simulink model "fft_core2"  (R2013a)
settings: Solver=VariableStepDiscrete  SolverMode=SingleTasking  StartTime=0.0  StopTime=4096*(4096/16) + 10000  RelTol=1e-3
undefined symbols (not defined in the file or in its folder): A, B, C, PCIN, xlipgetpartsetting
libraries: xbsIndex_r4 x20912, casper_library_misc x110, casper_library_reorder x8, casper_library_delays x4, xbsReplacements_r4 x2
(part 1 of 187)
settings Model: Creator=rprimian  LastModifiedBy=jack
settings Model: ModifiedComment=|
  | jack -- Wed Jan 14 18:05:02 2015 -- Version 1.207
  | resynthed
settings Model: ModifiedHistory=|
  | jack -- Wed Jan 14 18:05:02 2015 -- Version 1.207
  | resynthed
  | 
  | jack -- Wed Jan 14 17:38:02 2015 -- Version 1.206
  | 
  | 
  | jack -- Wed Jan 14 17:23:08 2015 -- Version 1.205
  | fanout write address / buf sel signals in unscrambler
  | 
  | jack -- Sun Jan 11 19:22:28 2015 -- Version 1.204
  | generated (lc off, equiv reg removal no)
  | 
  | jack -- Sun Jan 11 18:52:11 2015 -- Version 1.203
  | manual fanout control fft_stage_1 sync input
  | 
  | jack -- Sun Jan 11 12:56:59 2015 -- Version 1.202
  | regened
  | 
  | jack -- Sun Jan 11 12:38:07 2015 -- Version 1.201
  | manual fanout control between direct butterfly 2_0 and 3_0 sync
  | 
  | jack -- Sun Jan 11 12:11:23 2015 -- Version 1.200
  | implement counter in fft stage 1 as behavioural hdl
  | 
  | jack -- Fri Jan 09 10:07:59 2015 -- Version 1.199
  | generated
  | 
  | jack -- Wed Jan 07 15:06:47 2015 -- Version 1.198
  | xlupdatemodel for 14.7
  | 
  | jack -- Wed Jan 07 14:01:30 2015 -- Version 1.197
  | change butterfly max fanout to 2
  | 
  | jack -- Sun Dec 07 16:26:38 2014 -- Version 1.196
  | removed core delay attribute in coeff of butterfly 2_0
  | 
  | jack -- Thu Dec 04 23:51:50 2014 -- Version 1.195
  | change delay in butterfly 2-0 coeffgen to be core
  | 
  | jack -- Thu Dec 04 21:24:02 2014 -- Version 1.194
  | gen'd
  | 
  | jack -- Thu Dec 04 21:00:43 2014 -- Version 1.193
  | multiplexer latency=1
  | 
  | jack -- Wed Dec 03 18:09:45 2014 -- Version 1.192
  | regenerated
  | 
  | jack -- Wed Dec 03 15:44:47 2014 -- Version 1.191
  | regenerated
  | 
  | jack -- Wed Dec 03 14:18:08 2014 -- Version 1.190
  | added in descramble
  | 
  | jack -- Wed Dec 03 00:08:02 2014 -- Version 1.189
  | added back in butterfly2-0 sync out fanout regs
  | 
  | jack -- Tue Dec 02 21:40:43 2014 -- Version 1.188
  | all cast latency to 2 in fft direct
  | 
  | jack -- Tue Dec 02 17:31:35 2014 -- Version 1.187
  | remove input latency
  | 
  | jack -- Tue Dec 02 17:27:04 2014 -- Version 1.186
  | forgot to change hilbert addsubs to 'complex'
  | 
  | jack -- Tue Dec 02 17:16:05 2014 -- Version 1.185
  | ready to regenerate after fixing dsp complex adders and cmult latencies
  | 
  | jack -- Fri Nov 28 18:02:27 2014 -- Version 1.184
  | reduced fanout registering in cmult of butterfly 0_0 twiddle
  | 
  | jack -- Fri Nov 28 17:54:11 2014 -- Version 1.183
  | delay cores in biplex descramble reorder data delays
  | 
  | jack -- Fri Nov 28 17:51:35 2014 -- Version 1.182
  | implement sync delays in butterfly 3_0, 3_1 twiddles as cores
  | 
  | jack -- Fri Nov 28 15:14:09 2014 -- Version 1.181
  | regenerated
  | 
  | jack -- Fri Nov 28 14:47:31 2014 -- Version 1.180
  | update diagram
  | 
  | jack -- Fri Nov 28 14:11:29 2014 -- Version 1.179
  | 
  | syntax fix
  | 
  | jack -- Fri Nov 28 13:12:47 2014 -- Version 1.178
  | 
  | changed cast latency to 2 in both parts of FFT
  | 
  | jack -- Thu Nov 27 18:11:31 2014 -- Version 1.177
  | regenerated
  | 
  | jack -- Thu Nov 27 17:24:07 2014 -- Version 1.176
  | implement dsync 1 and dsync2 delays in fft stage 1 as cores (fanout control)
  | 
  | jack -- Wed Oct 29 13:45:38 2014 -- Version 1.175
  | regenerated in correct location
  | 
  | jack -- Wed Oct 29 08:59:41 2014 -- Version 1.174
  | wastn't generating to fft_core2.ngc! Last version of that file was from 26th oct 1159.
  | 
  | jack -- Wed Oct 29 02:01:36 2014 -- Version 1.173
  | 
  | 
  | jack -- Wed Oct 29 01:59:56 2014 -- Version 1.172
  | regenerated
  | 
  | jack -- Wed Oct 29 01:21:04 2014 -- Version 1.171
  | manual fanout control between direct butterfly 2_0 and 3_0 sync
  | 
  | jack -- Tue Oct 28 19:29:52 2014 -- Version 1.170
  | change latency between biplex and direct to 0
  | 
  | jack -- Mon Oct 27 18:43:05 2014 -- Version 1.169
  | added comment about manually changing hiltert addsubs to use dsp
  | 
  | jack -- Mon Oct 27 18:42:18 2014 -- Version 1.168
  | changed casts outside twiddles to latency 2, then redid manual changes
  | 
  | jack -- Sun Oct 26 11:03:45 2014 -- Version 1.167
  | dupe core for some experimenting :)
  | 
  | jack -- Sun Oct 26 10:45:07 2014 -- Version 1.166
  | delay on data-b in butterfly0_0 cmult changed to core
  | 
  | jack -- Sun Oct 26 10:25:39 2014 -- Version 1.165
  | latency between biplkex and direct back to 1
  | 
  | jack -- Sat Oct 25 15:09:40 2014 -- Version 1.164
  | regenerated
  | 
  | jack -- Sat Oct 25 14:36:46 2014 -- Version 1.163
  | do back to fabric adders in hilberts
  | 
  | jack -- Fri Oct 24 23:13:10 2014 -- Version 1.162
  | changed hilbert blocks in bi_real_unscr_4x to dsp implementation
  | 
  | jack -- Fri Oct 24 14:47:43 2014 -- Version 1.161
  | increased latency between biplex and direct fft to 2
  | 
  | jack -- Tue Oct 21 15:26:40 2014 -- Version 1.160
  | regenerated
  | 
  | jack -- Tue Oct 21 14:20:46 2014 -- Version 1.159
  | 
  | notes reminding me what to manually add if the FFT needs autmatically redrawing!
  | 
  | jack -- Tue Oct 21 14:18:23 2014 -- Version 1.158
  | 
  | made reorders in descramble not asynchronous
  | 
  | jack -- Tue Oct 21 11:02:41 2014 -- Version 1.157
  | 
  | 
  | jack -- Tue Oct 21 10:46:08 2014 -- Version 1.156
  | regenerated, after changing twiddle init script to reduce the number of fanout registers in cmults -- now it only puts a register where there is real fanout.
  | 
  | jack -- Tue Oct 21 09:44:16 2014 -- Version 1.155
  | 
  | 
  | jack -- Tue Oct 21 09:43:06 2014 -- Version 1.154
  | set dmux0 in fft_stage1 to use core delay (rather than behavioural HDL)
  | 
  | jack -- Mon Oct 20 17:21:54 2014 -- Version 1.153
  | generated
  | 
  | jack -- Mon Oct 20 15:57:34 2014 -- Version 1.152
  | remove channel order descramble
  | 
  | jack -- Mon Oct 20 15:47:10 2014 -- Version 1.150
  | 
  | change fft unscrambled to double buffer, and add some fanout delay. NOTE: this change requires manual setting of the FFT unscrambler block
  | 
  | jack -- Mon Oct 20 15:48:32 2014 -- Version 1.150
  | don't bother unscrambling
  | 
  | jack -- Mon Oct 20 10:32:55 2014 -- Version 1.149
  |  change data delays in bram_delay blocks to be inmplemented as cores. Reduce fanout delay from (max(1, log2(number_of_brams)) to max(1, log2(number_of_brams / max fanout))
  | 
  | jack -- Sun Oct 19 18:00:08 2014 -- Version 1.148
  | change add latency in biplex unscramble to 3, perform casts in xilinx cast blocks
  | 
  | jack -- Fri Oct 17 15:52:50 2014 -- Version 1.147
  | move adders everywhere to dsp. casts everywhere to logic
  | 
  | jack -- Wed Oct 15 14:23:41 2014 -- Version 1.146
  | regenerated with fft direct adders in dsps (one dsp per 2 adds / 2subs)
  | 
  | jack -- Wed Oct 15 11:45:00 2014 -- Version 1.145
  | 
  | changed fft direct to do adds in dsp. NOTE: This requires setting manually below the top level block!
  | 
  | jack -- Tue Oct 14 16:11:01 2014 -- Version 1.144
  | 
  | 
  | jack -- Mon Oct 13 18:35:49 2014 -- Version 1.143
  | redraw with 1 cycle latency on overflow comparators in butterflies
  | 
  | jack -- Thu Oct 09 14:59:23 2014 -- Version 1.142
  | regenerated
  | 
  | jack -- Thu Oct 09 14:39:22 2014 -- Version 1.141
  | replaced cmults with explicit dsp48 cmults using macros
  | 
  | jack -- Wed Oct 08 16:18:36 2014 -- Version 1.140
  | 
  | bram latency increase to 4 (only really necessary for the last stage of the dirrect butterflies, where there is no fanout and inadequate latency to go from bram to dsp in one clock)
  | 
  | jack -- Wed Oct 08 09:37:16 2014 -- Version 1.139
  | regenerated
  | 
  | jack -- Tue Oct 07 20:30:28 2014 -- Version 1.138
  | 
  | regnerated with cosin vanilla blocks in coefficient generators
  | 
  | jack -- Thu Sep 25 12:10:32 2014 -- Version 1.137
  | 
  | 
  | jack -- Thu Sep 25 12:10:01 2014 -- Version 1.136
  | 
  | 
  | jack -- Thu Sep 25 11:52:10 2014 -- Version 1.135
  | 
  | 
  | jack -- Thu Sep 25 10:42:48 2014 -- Version 1.134
  | 
  | manually changed the fft_unscrambler/reoder block.
  | -- double buffer
  | -- bram latency 3 (was 2)
  | -- manual drawing to fanout delay_sel and wr_addr signals
  | 
  | jack -- Tue Sep 23 10:03:49 2014 -- Version 1.133
  | 
  | synthesized
  | 
  | jack -- Mon Sep 22 14:47:38 2014 -- Version 1.132
  | changed adder implementation (in draw script) of butterfly adds to soft core (unless dsp chosen). Previously was behavioural
  | 
  | jack -- Sat Sep 20 12:31:03 2014 -- Version 1.131
  | 
  | compile (L shape constraints) failled spectacularly with dsp cast latency 2. Changed latency to 3.
  | Also lowered bram latency to 3
  | 
  | jack -- Fri Sep 19 18:08:32 2014 -- Version 1.130
  | regenerated
  | 
  | jack -- Fri Sep 19 15:47:10 2014 -- Version 1.129
  | 
  | changed cast latency in twiddles (which use dsps) to 2
  | 
  | jack -- Mon Sep 08 17:31:18 2014 -- Version 1.128
  | 
  | manual pipelining for fft_stage1
  | 
  | jack -- Tue Jun 03 23:16:33 2014 -- Version 1.127
  | 
  | 
  | jack -- Tue Jun 03 20:04:26 2014 -- Version 1.126
  | 
  | 
  | jack -- Mon Jun 02 09:04:22 2014 -- Version 1.125
  | pipelined overflow flag chain in fft direct
  | 
  | jack -- Mon Jun 02 07:25:10 2014 -- Version 1.124
  | manually added register stages to fft biplex stages 1 and 2.
  | changed convert latency in butterflies (dsp-based) to 4
  | 
  | jack -- Sat Mar 22 14:42:09 2014 -- Version 1.123
  | changed fft descramble to not use double buffering.
  | 
  | jack -- Fri Mar 21 17:47:36 2014 -- Version 1.122
  | changed reorder brams to optimize for speed
  | 
  | jack -- Sun Mar 16 21:17:26 2014 -- Version 1.121
  | fanout control on unscramblers
  | 
  | jack -- Thu Feb 20 17:09:35 2014 -- Version 1.120
  | changed bram latency in descramble to 3 to avoid using srls. will add more pipelineing in main model
  | 
  | jack -- Wed Feb 19 19:33:34 2014 -- Version 1.119
  | generated
  | 
  | jack -- Wed Feb 19 18:32:15 2014 -- Version 1.118
  | put bthe descramble back. changed max_fanout to 2
  | 
  | jack -- Fri Feb 14 17:39:39 2014 -- Version 1.117
  | 
  | 
  | jack -- Fri Feb 14 17:34:13 2014 -- Version 1.116
  | 
  | changed add latency to 3 (was 2) outside twiddles
  | 
  | jack -- Thu Feb 13 18:32:54 2014 -- Version 1.115
  | 
  | Easy timing fix to descramble -- don't bother doing it!
  | 
  | jack -- Thu Feb 13 18:11:13 2014 -- Version 1.114
  | 
  | turned down descramble bram latency to 3
  | 
  | jack -- Tue Feb 11 21:59:13 2014 -- Version 1.113
  | synth'd
  | 
  | jack -- Tue Feb 11 19:54:11 2014 -- Version 1.112
  | 
  | Changed brams in descramble reorder to optimize for speed
  | 
  | jack -- Tue Feb 11 17:12:22 2014 -- Version 1.111
  | 
  | Regenerated
  | 
  | jack -- Tue Feb 11 17:11:17 2014 -- Version 1.110
  | 
  | Changed reorder in fft_unscrambler to use double buffering, and fanout delay of 1
  | 
  | jack -- Tue Feb 04 10:57:01 2014 -- Version 1.109
  | regenerated
  | 
  | jack -- Mon Feb 03 17:18:37 2014 -- Version 1.108
  | change shift schedule
  | 
  | jack -- Mon Feb 03 13:02:14 2014 -- Version 1.107
  | complexified simulation outputs
  | 
  | jack -- Mon Feb 03 10:41:09 2014 -- Version 1.106
  | 
  | 
  | jack -- Mon Feb 03 10:39:20 2014 -- Version 1.105
  | 
  | 
  | jack -- Mon Feb 03 10:36:49 2014 -- Version 1.104
  | 
  | Added simulation model --  a series of 1 cycle impulsesat each of 4096 positions
  | 
  | jack -- Mon Feb 03 10:22:35 2014 -- Version 1.103
  | 
  | 
  | jack -- Sat Feb 01 23:42:24 2014 -- Version 1.102
  | Increased bram latency to 4
  | 
  | jack -- Fri Jan 31 22:38:23 2014 -- Version 1.101
  | 
  | Bug in fft_stage_n_init when using slice-based delays. A fanout delay was being compensated for on the sync lines, but did not actually appear on the data lines. Fixed this in the init script -- going for a recompile.
  | 
  | jack -- Fri Jan 31 17:45:46 2014 -- Version 1.100
  | 
  | Added a scope to input
  | 
  | jack -- Wed Jan 29 17:53:39 2014 -- Version 1.99
  | 
  | Generated core
  | 
  | jack -- Wed Jan 29 17:04:46 2014 -- Version 1.98
  | 
  | Changed max fanout to 1
  | 
  | jack -- Wed Jan 29 13:58:52 2014 -- Version 1.97
  | 
  | Changed delay blocks to attach constant 1 to we inputs. Before it was a constant going through a fanout/reinterpret/slice, which doesn't optimize away properly.
  | 
  | reverted to sampled constant one's. Failed compile with unsampled constants.
  | 
  | 
  | 
  | Recompile after setting we constants to be unsampled.
  | Previous compiles caused timing errors due to we fanout even though the signal is static
settings DataIOCC: SignalLoggingSaveFormat=ModelDataLogs
settings OptimizationCC: InlineParams=on  ExpressionDepthLimit=2147483647
settings DebuggingCC: FcnCallInpInsideContextMsg=UseLocalSettings
settings GRTTargetCC: CombineOutputUpdateFcns=off  GRTInterface=on

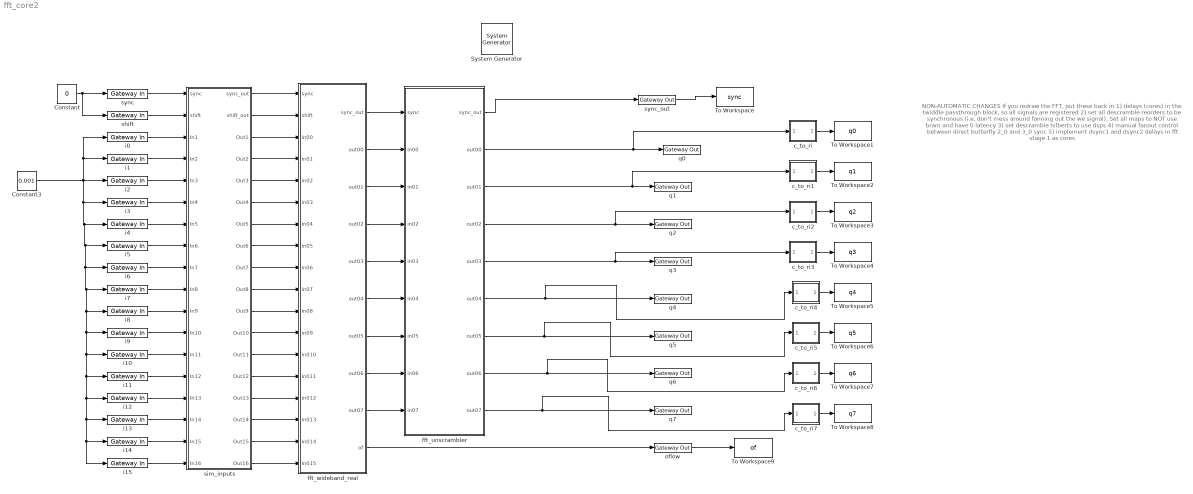
== system fft_core2 ==
  note: NON-AUTOMATIC CHANGES
      |
      | If you redraw the FFT, put these back in
      |
      | 1) delays (cores) in the twiddle passthrough block, so all signals are registered
      |
      | 2) set all descramble reorders to be synchronous (i.e, don't mess around fanning
      | out the we signal). Set all maps to NOT use bram and have 0 latency
      |
      | 3) set descramble hilberts to use dsps
      |
      | 4) manual fanout control between direct butterfly 2_0 and 3_0 sync
      |
      | 5) implement dsync1 and dsync2 delays in fft stage 1 as cores
  " System Generator" : xbsIndex_r4/ System Generator  Tag=genX  xilinxfamily=virtex6  part=xc6vsx475t  speed=-1  package=ff1759  synthesis_tool=XST  clock_wrapper=Clock Enables  directory=./fft_core2  proj_type=Project Navigator  Synth_file=XST Defaults  Impl_file=ISE Defaults  testbench=off  simulink_period=1  sysclk_period=3  dcm_input_clock_period=100  incr_netlist=off  trim_vbits=Everywhere in SubSystem  dbl_ovrd=According to Block Masks  core_generation=According to Block Masks  run_coregen=off  deprecated_control=off  eval_field=0  block_type=sysgen
      settings: block_version=11.4
  Constant : Constant  Value=0
  Constant3 : Constant  Value=0.001
  To Workspace : ToWorkspace  VariableName=sync  SampleTime=-1  SaveFormat=Timeseries
  To Workspace1 : ToWorkspace  VariableName=q0  SampleTime=-1  SaveFormat=Timeseries
  To Workspace2 : ToWorkspace  VariableName=q1  SampleTime=-1  SaveFormat=Timeseries
  To Workspace3 : ToWorkspace  VariableName=q2  SampleTime=-1  SaveFormat=Timeseries
  To Workspace4 : ToWorkspace  VariableName=q3  SampleTime=-1  SaveFormat=Timeseries
  To Workspace5 : ToWorkspace  VariableName=q4  SampleTime=-1  SaveFormat=Timeseries
  To Workspace6 : ToWorkspace  VariableName=q5  SampleTime=-1  SaveFormat=Timeseries
  To Workspace7 : ToWorkspace  VariableName=q6  SampleTime=-1  SaveFormat=Timeseries
  To Workspace8 : ToWorkspace  VariableName=q7  SampleTime=-1  SaveFormat=Timeseries
  To Workspace9 : ToWorkspace  VariableName=of  SampleTime=-1  SaveFormat=Timeseries
  c_to_ri : Subsystem
  c_to_ri1 : Subsystem
  c_to_ri2 : Subsystem
  c_to_ri3 : Subsystem
  c_to_ri4 : Subsystem
  c_to_ri5 : Subsystem
  c_to_ri6 : Subsystem
  c_to_ri7 : Subsystem
  fft_unscrambler : Subsystem  AncestorBlock=casper_library_ffts/fft_unscrambler  mask(fft_unscrambler){n_streams=1, FFTSize=11, n_inputs=3, n_bits_in=18, bram_latency=3, coeffs_bit_limit=8, async=off}
      mask prompts: n_streams "Number of simultaneous streams"; FFTSize "Size of FFT: (2^?)"; n_inputs "Number of simultaneous inputs: (2^?)"; n_bits_in "Input bit width"; bram_latency "BRAM Latency"; coeffs_bit_limit "Number bits above which to store map coefficients in BRAM (2^? bits)"; async "Asynchronous operation"
      mask init:
      | fft_unscrambler_init(gcb, ...
      |     'n_streams', n_streams, ...
      |     'FFTSize',FFTSize, ... 
      |     'n_inputs', n_inputs, ...
      |     'n_bits_in', n_bits_in, ...
      |     'bram_latency', bram_latency, ...
      |     'coeffs_bit_limit', coeffs_bit_limit, ...
      |     'async', async);
      settings: AttributesFormatString=FFTSize=11, n_inputs=3
  fft_wideband_real : Subsystem  Tag=casper:fft_wideband_real  AncestorBlock=casper_library_ffts/fft_wideband_real  mask(fft_wideband_real){n_streams=1, FFTSize=12, n_inputs=4, input_bit_width=18, bin_pt_in=17, coeff_bit_width=18, unscramble=off, async=off, add_latency=2, add_latency_twiddles=1, mult_latency=3, bram_latency=3, conv_latency=1, conv_latency_twiddles=1, input_latency=0, biplex_direct_latency=0, quantization=Round  (unbiased: +/- Inf), overflow=Wrap, delays_bit_limit=8, coeffs_bit_limit=8, coeff_sharing=off, coeff_decimation=off, coeff_generation=off, cal_bits=1, n_bits_rotation=25, mult_spec=1, max_fanout=4, bitgrowth=off, max_bits=19, hardcode_shifts=off, shift_schedule=[], dsp48_adders=on, conv_imp_twiddles=Xilinx Cast Block, conv_imp=Xilinx Cast Block}
      mask prompts: n_streams "Number simultaneous streams"; FFTSize "Size of FFT: (2^? pts)"; n_inputs "Number of Simultaneous Inputs: (2^?)"; input_bit_width "Input Bit Width"; bin_pt_in "Input binary point"; coeff_bit_width "Coefficient Bit Width"; unscramble "Unscramble output (ie, put channels in canonical order)"; async "Asynchronous operation"; add_latency "Add Latency"; add_latency_twiddles "Add Latency (in twiddles)"; mult_latency "Mult Latency"; bram_latency "BRAM Latency"; conv_latency "Convert Latency"; conv_latency_twiddles "Convert Latency (in twiddles)"; input_latency "Input Latency"; biplex_direct_latency "Latency between biplexes and fft_direct"; quantization "Quantization Behavior"; overflow "Overflow Behavior"; delays_bit_limit "Number bits above which to store stage's delays in BRAM (2^? bits)"; coeffs_bit_limit "Number bits above which to store stage's coefficients in BRAM (2^? bits)"; coeff_sharing "BRAM sharing in coeff storage"; coeff_decimation "Store a fraction of coeff factors where useful"; coeff_generation "Generate coeffs with multipliers where useful"; cal_bits "Number calibration locations when generating coeffs (2^?)"; n_bits_rotation "Feedback rotation vector resolution"; mult_spec "Multiplier impl. (0=core, 1=embedded, 2=behavioural) (left=1st stage, or just one value)"; max_fanout "Maximum fanout"; bitgrowth "Bitgrowth instead of shifting"; max_bits "Max bits to grow to"; hardcode_shifts "Hardcode shift schedule"; shift_schedule "Shift schedule"; dsp48_adders "DSP48 adders in butterfly"; conv_imp_twiddles "Convert implementation in twiddles"; conv_imp "Convert implementation elsewhere"
      mask help: A real-sampled wideband FFT.
      mask init:
      | fft_wideband_real_init(gcb, ...
      |     'n_streams', n_streams, ...
      |     'FFTSize', FFTSize, ...
      |     'n_inputs', n_inputs, ...
      |     'input_bit_width', input_bit_width, ...
      |     'bin_pt_in', bin_pt_in, ...
      |     'coeff_bit_width', coeff_bit_width, ...
      |     'unscramble', unscramble, ...
      |     'async', async, ...
      |     'add_latency', add_latency, ...
      |     'add_latency_twiddles', add_latency_twiddles, ...
      |     'mult_latency', mult_latency, ...
      |     'bram_latency', bram_latency, ...
      |     'conv_latency', conv_latency, ...
      |     'conv_latency_twiddles', conv_latency_twiddles, ...
      |     'input_latency', input_latency, ...
      |     'biplex_direct_latency', biplex_direct_latency, ...
      |     'quantization', quantization, ...
      |     'overflow', overflow, ...
      |     'delays_bit_limit', delays_bit_limit, ...
      |     'coeffs_bit_limit', coeffs_bit_limit, ...
      |     'coeff_sharing', coeff_sharing, ...
      |     'coeff_decimation', coeff_decimation, ...
      |     'coeff_generation', coeff_generation, ...
      |     'cal_bits', cal_bits, ...
      |     'n_bits_rotation', n_bits_rotation, ...
      |     'max_fanout', max_fanout, ...   
      |     'mult_spec', mult_spec, ...
      |     'bitgrowth', bitgrowth, ...
      |     'max_bits', max_bits, ...
      |     'hardcode_shifts', hardcode_shifts, ...
      |     'shift_schedule', shift_schedule, ...
      |     'dsp48_adders', dsp48_adders, ...
      |     'conv_imp_twiddles', conv_imp_twiddles, ...
      |     'conv_imp', conv_imp);
      settings: AttributesFormatString=|
      | 12 stages
      | (18,18)
      | Round  (unbiased: +/- Inf)
      | Wrap
      mask Help: eval('xlWeb(''http://casper.berkeley.edu/wiki/Fft_wideband_real'')')
      mask TypeOptions quantization: Truncate | Round  (unbiased: +/- Inf) | Round  (unbiased: Even Values)
      mask TypeOptions overflow: Wrap | Saturate | Error
      mask Callback hardcode_shifts:
      | hardcode_shifts = get_param(gcb, 'hardcode_shifts');
      | set_param_state(gcb, 'shift_schedule', hardcode_shifts);
      mask Callback dsp48_adders: fft_callback_dsp48_adders(gcb);
      mask TypeOptions conv_imp_twiddles: Fabric | DSP48 | Behavioural | Xilinx Cast Block
      mask TypeOptions conv_imp: Fabric | DSP48 | Behavioural | Xilinx Cast Block
  i{0..15} (16 alike) : xbsIndex_r4/Gateway In  gui_display_data_type=Fixed-point  arith_type="Signed  (2's comp)"  n_bits=18  bin_pt=17  preci_type=Single  exp_width=8  frac_width=24  quantization="Round  (unbiased: +/- Inf)"  overflow=Saturate  period=1  dbl_ovrd=off  timing_constraint=None  locs_specified=off  LOCs={}  UseAsADC=off  ADCChannel='1'  inherit_from_input=off  hdl_port=on  block_type=gatewayin
      settings: infoedit="Gateway in block.  Converts inputs of type Simulink integer, double and fixed point to  Xilinx fixed point type.<br><br>Hardware notes:  In hardware these blocks become top level input ports."  block_version=11.4
  oflow : xbsIndex_r4/Gateway Out  inherit_from_input=on  hdl_port=on  timing_constraint=None  locs_specified=off  LOCs={}  UseAsDAC=off  DACChannel='1'  block_type=gatewayout
      settings: block_version=11.4
  q{0..7} (8 alike) : xbsIndex_r4/Gateway Out  inherit_from_input=on  hdl_port=on  timing_constraint=None  locs_specified=off  LOCs={}  UseAsDAC=off  DACChannel='1'  block_type=gatewayout
      settings: block_version=11.4
  shift : xbsIndex_r4/Gateway In  gui_display_data_type=Fixed-point  arith_type=Unsigned  n_bits=15  bin_pt=0  preci_type=Single  exp_width=8  frac_width=24  quantization="Round  (unbiased: +/- Inf)"  overflow=Saturate  period=1  dbl_ovrd=off  timing_constraint=None  locs_specified=off  LOCs={}  UseAsADC=off  ADCChannel='1'  inherit_from_input=off  hdl_port=on  block_type=gatewayin
      settings: infoedit="Gateway in block.  Converts inputs of type Simulink integer, double and fixed point to  Xilinx fixed point type.<br><br>Hardware notes:  In hardware these blocks become top level input ports."  block_version=11.4
  sim_inputs : Subsystem
  sync : xbsIndex_r4/Gateway In  gui_display_data_type=Fixed-point  arith_type=Boolean  n_bits=1  bin_pt=0  preci_type=Single  exp_width=8  frac_width=24  quantization="Round  (unbiased: +/- Inf)"  overflow=Saturate  period=1  dbl_ovrd=off  timing_constraint=None  locs_specified=off  LOCs={}  UseAsADC=off  ADCChannel='1'  inherit_from_input=off  hdl_port=on  block_type=gatewayin
      settings: infoedit="Gateway in block.  Converts inputs of type Simulink integer, double and fixed point to  Xilinx fixed point type.<br><br>Hardware notes:  In hardware these blocks become top level input ports."  block_version=11.4
  sync_out : xbsIndex_r4/Gateway Out  inherit_from_input=on  hdl_port=on  timing_constraint=None  locs_specified=off  LOCs={}  UseAsDAC=off  DACChannel='1'  block_type=gatewayout
      settings: block_version=11.4
  wires:
  Constant/1 -> sync/1, shift/1
  fft_wideband_real/1(sync_out) -> fft_unscrambler/1(sync)
  fft_wideband_real/2(out00) -> fft_unscrambler/2(in00)
  fft_wideband_real/3(out01) -> fft_unscrambler/3(in01)
  fft_wideband_real/4(out02) -> fft_unscrambler/4(in02)
  fft_wideband_real/5(out03) -> fft_unscrambler/5(in03)
  fft_wideband_real/6(out04) -> fft_unscrambler/6(in04)
  fft_wideband_real/7(out05) -> fft_unscrambler/7(in05)
  fft_wideband_real/8(out06) -> fft_unscrambler/8(in06)
  fft_wideband_real/9(out07) -> fft_unscrambler/9(in07)
  fft_wideband_real/10(of) -> oflow/1
  Constant3/1 -> i0/1, i1/1, i15/1, i14/1, i13/1, i12/1, i11/1, i10/1, i9/1, i8/1, i7/1, i6/1, i5/1, i4/1, i3/1, i2/1
  sync_out/1 -> To Workspace/1
  shift/1 -> sim_inputs/2(shift)
  sync/1 -> sim_inputs/1(sync)
  i9/1 -> sim_inputs/12(In10)
  i8/1 -> sim_inputs/11(In9)
  i7/1 -> sim_inputs/10(In8)
  i6/1 -> sim_inputs/9(In7)
  i5/1 -> sim_inputs/8(In6)
  i3/1 -> sim_inputs/6(In4)
  i4/1 -> sim_inputs/7(In5)
  i15/1 -> sim_inputs/18(In16)
  i2/1 -> sim_inputs/5(In3)
  i14/1 -> sim_inputs/17(In15)
  i13/1 -> sim_inputs/16(In14)
  i12/1 -> sim_inputs/15(In13)
  i11/1 -> sim_inputs/14(In12)
  i10/1 -> sim_inputs/13(In11)
  i1/1 -> sim_inputs/4(In2)
  i0/1 -> sim_inputs/3(In1)
  sim_inputs/12(Out10) -> fft_wideband_real/12(in09)
  sim_inputs/10(Out8) -> fft_wideband_real/10(in07)
  sim_inputs/14(Out12) -> fft_wideband_real/14(in011)
  sim_inputs/11(Out9) -> fft_wideband_real/11(in08)
  sim_inputs/17(Out15) -> fft_wideband_real/17(in014)
  sim_inputs/6(Out4) -> fft_wideband_real/6(in03)
  sim_inputs/15(Out13) -> fft_wideband_real/15(in012)
  sim_inputs/7(Out5) -> fft_wideband_real/7(in04)
  sim_inputs/13(Out11) -> fft_wideband_real/13(in010)
  sim_inputs/3(Out1) -> fft_wideband_real/3(in00)
  sim_inputs/8(Out6) -> fft_wideband_real/8(in05)
  sim_inputs/9(Out7) -> fft_wideband_real/9(in06)
  sim_inputs/1(sync_out) -> fft_wideband_real/1(sync)
  sim_inputs/16(Out14) -> fft_wideband_real/16(in013)
  sim_inputs/2(shift_out) -> fft_wideband_real/2(shift)
  sim_inputs/4(Out2) -> fft_wideband_real/4(in01)
  sim_inputs/18(Out16) -> fft_wideband_real/18(in015)
  sim_inputs/5(Out3) -> fft_wideband_real/5(in02)
  c_to_ri/1(Out1) -> To Workspace1/1
  c_to_ri1/1(Out1) -> To Workspace2/1
  c_to_ri2/1(Out1) -> To Workspace3/1
  c_to_ri3/1(Out1) -> To Workspace4/1
  c_to_ri4/1(Out1) -> To Workspace5/1
  c_to_ri5/1(Out1) -> To Workspace6/1
  c_to_ri6/1(Out1) -> To Workspace7/1
  c_to_ri7/1(Out1) -> To Workspace8/1
  oflow/1 -> To Workspace9/1
  fft_unscrambler/1(sync_out) -> sync_out/1
  fft_unscrambler/2(out00) -> c_to_ri/1(In1), q0/1
  fft_unscrambler/3(out01) -> c_to_ri1/1(In1), q1/1
  fft_unscrambler/4(out02) -> c_to_ri2/1(In1), q2/1
  fft_unscrambler/5(out03) -> c_to_ri3/1(In1), q3/1
  fft_unscrambler/6(out04) -> c_to_ri4/1(In1), q4/1
  fft_unscrambler/7(out05) -> c_to_ri5/1(In1), q5/1
  fft_unscrambler/8(out06) -> c_to_ri6/1(In1), q6/1
  fft_unscrambler/9(out07) -> c_to_ri7/1(In1), q7/1

== system fft_core2/c_to_ri ==
  In1 : Inport
  Real-Imag to Complex : RealImagToComplex
  c_to_ri : casper_library_misc/c_to_ri  n_bits=18  bin_pt=17
  r : xbsIndex_r4/Gateway Out  inherit_from_input=off  hdl_port=off  timing_constraint=None  locs_specified=off  LOCs={}  UseAsDAC=off  DACChannel='1'  block_type=gatewayout
      settings: block_version=11.4
  r1 : xbsIndex_r4/Gateway Out  inherit_from_input=off  hdl_port=off  timing_constraint=None  locs_specified=off  LOCs={}  UseAsDAC=off  DACChannel='1'  block_type=gatewayout
      settings: block_version=11.4
  Out1 : Outport
  wires:
  c_to_ri/2 -> r1/1
  Real-Imag to Complex/1 -> Out1/1
  r/1 -> Real-Imag to Complex/1
  c_to_ri/1 -> r/1
  r1/1 -> Real-Imag to Complex/2
  In1/1 -> c_to_ri/1

== system fft_core2/c_to_ri1 ==
  In1 : Inport
  Real-Imag to Complex : RealImagToComplex
  c_to_ri : casper_library_misc/c_to_ri  n_bits=18  bin_pt=17
  r : xbsIndex_r4/Gateway Out  inherit_from_input=off  hdl_port=off  timing_constraint=None  locs_specified=off  LOCs={}  UseAsDAC=off  DACChannel='1'  block_type=gatewayout
      settings: block_version=11.4
  r1 : xbsIndex_r4/Gateway Out  inherit_from_input=off  hdl_port=off  timing_constraint=None  locs_specified=off  LOCs={}  UseAsDAC=off  DACChannel='1'  block_type=gatewayout
      settings: block_version=11.4
  Out1 : Outport
  wires:
  In1/1 -> c_to_ri/1
  r1/1 -> Real-Imag to Complex/2
  c_to_ri/1 -> r/1
  r/1 -> Real-Imag to Complex/1
  Real-Imag to Complex/1 -> Out1/1
  c_to_ri/2 -> r1/1

== system fft_core2/c_to_ri2 ==
  In1 : Inport
  Real-Imag to Complex : RealImagToComplex
  c_to_ri : casper_library_misc/c_to_ri  n_bits=18  bin_pt=17
  r : xbsIndex_r4/Gateway Out  inherit_from_input=off  hdl_port=off  timing_constraint=None  locs_specified=off  LOCs={}  UseAsDAC=off  DACChannel='1'  block_type=gatewayout
      settings: block_version=11.4
  r1 : xbsIndex_r4/Gateway Out  inherit_from_input=off  hdl_port=off  timing_constraint=None  locs_specified=off  LOCs={}  UseAsDAC=off  DACChannel='1'  block_type=gatewayout
      settings: block_version=11.4
  Out1 : Outport
  wires:
  In1/1 -> c_to_ri/1
  r1/1 -> Real-Imag to Complex/2
  c_to_ri/1 -> r/1
  r/1 -> Real-Imag to Complex/1
  Real-Imag to Complex/1 -> Out1/1
  c_to_ri/2 -> r1/1

== system fft_core2/c_to_ri3 ==
  In1 : Inport
  Real-Imag to Complex : RealImagToComplex
  c_to_ri : casper_library_misc/c_to_ri  n_bits=18  bin_pt=17
  r : xbsIndex_r4/Gateway Out  inherit_from_input=off  hdl_port=off  timing_constraint=None  locs_specified=off  LOCs={}  UseAsDAC=off  DACChannel='1'  block_type=gatewayout
      settings: block_version=11.4
  r1 : xbsIndex_r4/Gateway Out  inherit_from_input=off  hdl_port=off  timing_constraint=None  locs_specified=off  LOCs={}  UseAsDAC=off  DACChannel='1'  block_type=gatewayout
      settings: block_version=11.4
  Out1 : Outport
  wires:
  c_to_ri/2 -> r1/1
  Real-Imag to Complex/1 -> Out1/1
  r/1 -> Real-Imag to Complex/1
  c_to_ri/1 -> r/1
  r1/1 -> Real-Imag to Complex/2
  In1/1 -> c_to_ri/1

== system fft_core2/c_to_ri4 ==
  In1 : Inport
  Real-Imag to Complex : RealImagToComplex
  c_to_ri : casper_library_misc/c_to_ri  n_bits=18  bin_pt=17
  r : xbsIndex_r4/Gateway Out  inherit_from_input=off  hdl_port=off  timing_constraint=None  locs_specified=off  LOCs={}  UseAsDAC=off  DACChannel='1'  block_type=gatewayout
      settings: block_version=11.4
  r1 : xbsIndex_r4/Gateway Out  inherit_from_input=off  hdl_port=off  timing_constraint=None  locs_specified=off  LOCs={}  UseAsDAC=off  DACChannel='1'  block_type=gatewayout
      settings: block_version=11.4
  Out1 : Outport
  wires:
  In1/1 -> c_to_ri/1
  r1/1 -> Real-Imag to Complex/2
  c_to_ri/1 -> r/1
  r/1 -> Real-Imag to Complex/1
  Real-Imag to Complex/1 -> Out1/1
  c_to_ri/2 -> r1/1

== system fft_core2/c_to_ri5 ==
  In1 : Inport
  Real-Imag to Complex : RealImagToComplex
  c_to_ri : casper_library_misc/c_to_ri  n_bits=18  bin_pt=17
  r : xbsIndex_r4/Gateway Out  inherit_from_input=off  hdl_port=off  timing_constraint=None  locs_specified=off  LOCs={}  UseAsDAC=off  DACChannel='1'  block_type=gatewayout
      settings: block_version=11.4
  r1 : xbsIndex_r4/Gateway Out  inherit_from_input=off  hdl_port=off  timing_constraint=None  locs_specified=off  LOCs={}  UseAsDAC=off  DACChannel='1'  block_type=gatewayout
      settings: block_version=11.4
  Out1 : Outport
  wires:
  c_to_ri/2 -> r1/1
  Real-Imag to Complex/1 -> Out1/1
  r/1 -> Real-Imag to Complex/1
  c_to_ri/1 -> r/1
  r1/1 -> Real-Imag to Complex/2
  In1/1 -> c_to_ri/1

== system fft_core2/c_to_ri6 ==
  In1 : Inport
  Real-Imag to Complex : RealImagToComplex
  c_to_ri : casper_library_misc/c_to_ri  n_bits=18  bin_pt=17
  r : xbsIndex_r4/Gateway Out  inherit_from_input=off  hdl_port=off  timing_constraint=None  locs_specified=off  LOCs={}  UseAsDAC=off  DACChannel='1'  block_type=gatewayout
      settings: block_version=11.4
  r1 : xbsIndex_r4/Gateway Out  inherit_from_input=off  hdl_port=off  timing_constraint=None  locs_specified=off  LOCs={}  UseAsDAC=off  DACChannel='1'  block_type=gatewayout
      settings: block_version=11.4
  Out1 : Outport
  wires:
  c_to_ri/2 -> r1/1
  Real-Imag to Complex/1 -> Out1/1
  r/1 -> Real-Imag to Complex/1
  c_to_ri/1 -> r/1
  r1/1 -> Real-Imag to Complex/2
  In1/1 -> c_to_ri/1

== system fft_core2/c_to_ri7 ==
  In1 : Inport
  Real-Imag to Complex : RealImagToComplex
  c_to_ri : casper_library_misc/c_to_ri  n_bits=18  bin_pt=17
  r : xbsIndex_r4/Gateway Out  inherit_from_input=off  hdl_port=off  timing_constraint=None  locs_specified=off  LOCs={}  UseAsDAC=off  DACChannel='1'  block_type=gatewayout
      settings: block_version=11.4
  r1 : xbsIndex_r4/Gateway Out  inherit_from_input=off  hdl_port=off  timing_constraint=None  locs_specified=off  LOCs={}  UseAsDAC=off  DACChannel='1'  block_type=gatewayout
      settings: block_version=11.4
  Out1 : Outport
  wires:
  In1/1 -> c_to_ri/1
  r1/1 -> Real-Imag to Complex/2
  c_to_ri/1 -> r/1
  r/1 -> Real-Imag to Complex/1
  Real-Imag to Complex/1 -> Out1/1
  c_to_ri/2 -> r1/1
